simulink model "MSDR_v1"  (R2018a)
settings: Solver=ode23tb  StartTime=0.0  StopTime=50000  RelTol=1e-3
values from neighbouring files (symbols this model uses):
  a_f = -3.22E-5    (= -3.22e-05)    [MSDR_parameters.m]
  a_g = +2.35E-5    (= 2.35e-05)    [MSDR_parameters.m]
  beta = [0.000223, 0.001457, 0.001307, 0.002628, 0.000766, 0.000280]    [MSDR_parameters.m]
  beta_t = sum(beta)    [MSDR_parameters.m]
  Cp_s_shx = 1549.12e-6    (= 0.00154912)    [MSDR_parameters.m]
  Cst = 10    [MSDR_parameters.m]
  dLb = 0    [MSDR_parameters.m]
  dLs = 0    [MSDR_parameters.m]
  dLsc = 0    [MSDR_parameters.m]
  gamma_I = 5.1135e-2    (= 0.051135)    [MSDR_parameters.m]
  gamma_Xe = 1.1628e-2    (= 0.011628)    [MSDR_parameters.m]
  hA_fg = [h_fg*A_fg/2, h_fg*A_fg/2]    [MSDR_parameters.m]
  hA_p_phx1 = h_p_phx*A_p_phx    [MSDR_parameters.m]
  hA_p_phx2 = h_p_phx*A_p_phx    [MSDR_parameters.m]
  hA_p_phx3 = h_p_phx*A_p_phx    [MSDR_parameters.m]
  hA_p_phx4 = h_p_phx*A_p_phx    [MSDR_parameters.m]
  hA_p_phx5 = h_p_phx*A_p_phx    [MSDR_parameters.m]
  hA_p_phx6 = h_p_phx*A_p_phx    [MSDR_parameters.m]
  hA_p_shx1 = h_p_shx*A_p_shx    [MSDR_parameters.m]
  hA_p_shx2 = h_p_shx*A_p_shx    [MSDR_parameters.m]
  hA_p_shx3 = h_p_shx*A_p_shx    [MSDR_parameters.m]
  hA_p_shx4 = h_p_shx*A_p_shx    [MSDR_parameters.m]
  hA_p_shx5 = h_p_shx*A_p_shx    [MSDR_parameters.m]
  hA_p_shx6 = h_p_shx*A_p_shx    [MSDR_parameters.m]
  hA_s_phx1 = h_s_phx*A_s_phx    [MSDR_parameters.m]
  hA_s_phx2 = h_s_phx*A_s_phx    [MSDR_parameters.m]
  hA_s_phx3 = h_s_phx*A_s_phx    [MSDR_parameters.m]
  hA_s_phx4 = h_s_phx*A_s_phx    [MSDR_parameters.m]
  hA_s_phx5 = h_s_phx*A_s_phx    [MSDR_parameters.m]
  hA_s_phx6 = h_s_phx*A_s_phx    [MSDR_parameters.m]
  hA_s_shx1 = h_s_shx*A_s_shx    [MSDR_parameters.m]
  hA_s_shx2 = h_s_shx*A_s_shx    [MSDR_parameters.m]
  hA_s_shx3 = h_s_shx*A_s_shx    [MSDR_parameters.m]
  hA_s_shx4 = h_s_shx*A_s_shx    [MSDR_parameters.m]
  hA_s_shx5 = h_s_shx*A_s_shx    [MSDR_parameters.m]
  hA_s_shx6 = h_s_shx*A_s_shx    [MSDR_parameters.m]
  I_0 = gamma_I*Sig_f_msdr*phi_0/lam_I    (= 4.38204721773e+16)    [MSDR_parameters.m]
  Ifa = [0.25, 0.25]    [MSDR_parameters.m]
  Ifb = [0.25, 0.25]    [MSDR_parameters.m]
  Ig = [0.5, 0.5]    [MSDR_parameters.m]
  J = 1e-6    (= 1e-06)    [MSDR_parameters.m]
  ka = [0.235, 0.235]    [MSDR_parameters.m]
  kb = [0.235, 0.235]    [MSDR_parameters.m]
  kc = 5    [MSDR_parameters.m]
  kga = [0.015, 0.015]    [MSDR_parameters.m]
  kgb = [0.015, 0.015]    [MSDR_parameters.m]
  L = 8.5344    [MSDR_parameters.m]
  Lam = 2.400E-04    (= 0.00024)    [MSDR_parameters.m]
  lam = [0.0124, 0.0305, 0.111, 0.301, 1.14, 3.01]    [MSDR_parameters.m]
  lam_bubl = 2.0e-2    (= 0.02)    [MSDR_parameters.m]
  lam_I = 2.875e-5    (= 2.875e-05)    [MSDR_parameters.m]
  lam_Xe = 2.0916e-5    (= 2.0916e-05)    [MSDR_parameters.m]
  m_3m = W_3*2    (= 8618.207327)    [MSDR_parameters.m]
  m_fm = W_f*2    (= 9978.96)    [MSDR_parameters.m]
  m_sb = 1717    [MSDR_parameters.m]
  mb_cpb = 2.689619410657651e+00    (= 2.68961941066)    [MSDR_parameters.m]
  mcp_fa = mfa*Cp_f    [MSDR_parameters.m]
  mcp_fb = mfb*Cp_f    [MSDR_parameters.m]
  mcp_g = mg*Cp_g    [MSDR_parameters.m]
  mcp_p_phx1 = Cp_p_phx*mp_phx1    [MSDR_parameters.m]
  mcp_p_phx2 = Cp_p_phx*mp_phx2    [MSDR_parameters.m]
  mcp_p_phx3 = Cp_p_phx*mp_phx3    [MSDR_parameters.m]
  mcp_p_phx4 = Cp_p_phx*mp_phx4    [MSDR_parameters.m]
  mcp_p_phx5 = Cp_p_phx*mp_phx5    [MSDR_parameters.m]
  mcp_p_phx6 = Cp_p_phx*mp_phx6    [MSDR_parameters.m]
  mcp_p_shx1 = Cp_p_shx*mp_shx1    [MSDR_parameters.m]
  mcp_p_shx2 = Cp_p_shx*mp_shx2    [MSDR_parameters.m]
  mcp_p_shx3 = Cp_p_shx*mp_shx3    [MSDR_parameters.m]
  mcp_p_shx4 = Cp_p_shx*mp_shx4    [MSDR_parameters.m]
  mcp_p_shx5 = Cp_p_shx*mp_shx5    [MSDR_parameters.m]
  mcp_p_shx6 = Cp_p_shx*mp_shx6    [MSDR_parameters.m]
  mcp_s_phx1 = Cp_s_phx*ms_phx1    [MSDR_parameters.m]
  mcp_s_phx2 = Cp_s_phx*ms_phx2    [MSDR_parameters.m]
  mcp_s_phx3 = Cp_s_phx*ms_phx3    [MSDR_parameters.m]
  mcp_s_phx4 = Cp_s_phx*ms_phx4    [MSDR_parameters.m]
  mcp_s_phx5 = Cp_s_phx*ms_phx5    [MSDR_parameters.m]
  mcp_s_phx6 = Cp_s_phx*ms_phx6    [MSDR_parameters.m]
  mcp_s_shx1 = Cp_s_shx*ms_shx1    [MSDR_parameters.m]
  mcp_s_shx2 = Cp_s_shx*ms_shx1    [MSDR_parameters.m]
  mcp_s_shx3 = Cp_s_shx*ms_shx1    [MSDR_parameters.m]
  mcp_s_shx4 = Cp_s_shx*ms_shx1    [MSDR_parameters.m]
  mcp_s_shx5 = Cp_s_shx*ms_shx1    [MSDR_parameters.m]
  mcp_s_shx6 = Cp_s_shx*ms_shx1    [MSDR_parameters.m]
  mcp_t_phx1 = Cp_t_phx*mt_phx1    [MSDR_parameters.m]
  mcp_t_phx2 = Cp_t_phx*mt_phx2    [MSDR_parameters.m]
  mcp_t_phx3 = Cp_t_phx*mt_phx3    [MSDR_parameters.m]
  mcp_t_phx4 = Cp_t_phx*mt_phx4    [MSDR_parameters.m]
  mcp_t_phx5 = Cp_t_phx*mt_phx5    [MSDR_parameters.m]
  mcp_t_phx6 = Cp_t_phx*mt_phx6    [MSDR_parameters.m]
  mcp_t_shx1 = Cp_t_phx*mt_shx1    [MSDR_parameters.m]
  mcp_t_shx2 = Cp_t_phx*mt_shx2    [MSDR_parameters.m]
  mcp_t_shx3 = Cp_t_phx*mt_shx3    [MSDR_parameters.m]
  mcp_t_shx4 = Cp_t_phx*mt_shx4    [MSDR_parameters.m]
  mcp_t_shx5 = Cp_t_phx*mt_shx5    [MSDR_parameters.m]
  mcp_t_shx6 = Cp_t_phx*mt_shx6    [MSDR_parameters.m]
  mfa = [mass_fn, mass_fn]    [MSDR_parameters.m]
  mfb = [mass_fn, mass_fn]    [MSDR_parameters.m]
  mp_phx1 = [494.7, 494.7, 494.7, 494.7]    [MSDR_parameters.m]
  mp_phx2 = [494.7, 494.7, 494.7, 494.7]    [MSDR_parameters.m]
  mp_phx3 = [494.7, 494.7, 494.7, 494.7]    [MSDR_parameters.m]
  mp_phx4 = [494.7, 494.7, 494.7, 494.7]    [MSDR_parameters.m]
  mp_phx5 = [494.7, 494.7, 494.7, 494.7]    [MSDR_parameters.m]
  mp_phx6 = [494.7, 494.7, 494.7, 494.7]    [MSDR_parameters.m]
  mp_phxm = (Wp_phx1 + Wp_phx2)*1    (= 1663.16)    [MSDR_parameters.m]
  mp_shx1 = [429.3, 429.3, 429.3, 429.3]    [MSDR_parameters.m]
  mp_shx2 = [429.3, 429.3, 429.3, 429.3]    [MSDR_parameters.m]
  mp_shx3 = [429.3, 429.3, 429.3, 429.3]    [MSDR_parameters.m]
  mp_shx4 = [429.3, 429.3, 429.3, 429.3]    [MSDR_parameters.m]
  mp_shx5 = [429.3, 429.3, 429.3, 429.3]    [MSDR_parameters.m]
  mp_shx6 = [429.3, 429.3, 429.3, 429.3]    [MSDR_parameters.m]
  mp_shxm = (Wp_shx1 + Wp_shx2)*1    (= 932.38)    [MSDR_parameters.m]
  ms_phx1 = [1152.5, 1152.5, 1152.5, 1152.5]    [MSDR_parameters.m]
  ms_phx2 = [1152.5, 1152.5, 1152.5, 1152.5]    [MSDR_parameters.m]
  ms_phx3 = [1152.5, 1152.5, 1152.5, 1152.5]    [MSDR_parameters.m]
  ms_phx4 = [1152.5, 1152.5, 1152.5, 1152.5]    [MSDR_parameters.m]
  ms_phx5 = [1152.5, 1152.5, 1152.5, 1152.5]    [MSDR_parameters.m]
  ms_phx6 = [1152.5, 1152.5, 1152.5, 1152.5]    [MSDR_parameters.m]
  ms_phxm = (Ws_phx1 + Ws_phx2)*1    (= 932.38)    [MSDR_parameters.m]
  ms_shx1 = [1861.5, 1861.5, 1861.5, 1861.5]    [MSDR_parameters.m]
  ms_shx2 = [1861.5, 1861.5, 1861.5, 1861.5]    [MSDR_parameters.m]
  ... (+104 more)
undefined symbols (not defined in the file or in its folder): Ak2, As, C0, Cpp, Cps, Cpsc, Cpw, Dit, Dot, hA_p_thx1, hA_p_thx2, hA_p_thx3, hA_s_thx1, hA_s_thx2, hA_s_thx3, hc0, hfg, hfw0, HFW1, hfw10, HFW2, hpw, Hr, hr0, hwb, hws, hwsc, K3, KBHP, KBLP, Lsc, mcp_p_thx1, mcp_p_thx2, mcp_p_thx3, mcp_s_thx1, mcp_s_thx2, mcp_s_thx3, mcp_t_thx1, mcp_t_thx2, mcp_t_thx3, mp_thx1, mp_thx2, mp_thx3, ms_thx1, ms_thx2, ms_thx3, Mstm, nuf, Pp2, Pp3, Pp4, Pp5
libraries: simulink x20, aerolibconvert2 x2
(part 4 of 7)

== system MSDR_v1/HEAT EXCHANGERS/HEAT EXCHANGER LOOP 2/PHX3 HEAT TRANSFER ==
  PRIMARY FLUID INLET TEMPERATURE : Inport
  SECONDARY FLUID INLET TEMPERATURE : Inport  Port=2
  PRIMARY FLOW FRACTION : Inport  Port=3
  PRIMARY HEAT TRANSFER FRACTION : Inport  Port=4
  SECONDARY FLOW FRACTION : Inport  Port=5
  SECONDARY HEAT TRANSFER FRACTION : Inport  Port=6
  Mux : Mux  Inputs=16
      settings: DisplayOption=signals
  To Workspace : ToWorkspace  VariableName=phx3_ht  SampleTime=-1
  Tp1_phx3 : Integrator  InitialCondition=T0_p_phx3(1)
  Tp2_phx3 : Integrator  InitialCondition=T0_p_phx3(2)
  "Tp3_phx3 " : Integrator  InitialCondition=T0_p_phx3(3)
  Tp4_phx3 : Integrator  InitialCondition=T0_p_phx3(4)
  Ts1_phx3 : Integrator  InitialCondition=T0_s_phx3(1)
  Ts2_phx3 : Integrator  InitialCondition=T0_s_phx3(2)
  Ts3_phx3 : Integrator  InitialCondition=T0_s_phx3(3)
  Ts4_phx3 : Integrator  InitialCondition=T0_s_phx3(4)
  Tt1_phx3 : Integrator  InitialCondition=T0_t_phx3(1)
  Tt2_phx3 : Integrator  InitialCondition=T0_t_phx3(2)
  d(Tp1_phx3)/dt : Fcn  Expr=(u[13]*Wp_phx3/mp_phx3(1))*(u[1] - u[3]) + (u[14]*hA_p_phx3(1)/mcp_p_phx3(1))*(u[7] - u[3])
  d(Tp2_phx3)/dt : Fcn  Expr=(u[13]*Wp_phx3/mp_phx3(2))*(u[3] - u[4]) + (u[14]*hA_p_phx3(2)/mcp_p_phx3(2))*(u[7] - u[3])
  d(Tp3_phx3)/dt : Fcn  Expr=(u[13]*Wp_phx3/mp_phx3(3))*(u[4] - u[5]) + (u[14]*hA_p_phx3(3)/mcp_p_phx3(3))*(u[8] - u[5])
  d(Tp4_phx3)/dt : Fcn  Expr=(u[13]*Wp_phx3/mp_phx3(4))*(u[5] - u[6]) + (u[14]*hA_p_phx3(4)/mcp_p_phx3(4))*(u[8] - u[5])
  d(Ts1_phx3)/dt : Fcn  Expr=(u[15]*Ws_phx3/ms_phx3(1))*(u[2] - u[9]) + (u[16]*hA_s_phx3(1)/mcp_s_phx3(1))*(u[8] - u[9])
  d(Ts2_phx3)/dt : Fcn  Expr=(u[15]*Ws_phx3/ms_phx3(2))*(u[9] - u[10]) + (u[16]*hA_s_phx3(2)/mcp_s_phx3(2))*(u[8] - u[9])
  d(Ts3_phx3)/dt : Fcn  Expr=(u[15]*Ws_phx3/ms_phx3(3))*(u[10] - u[11]) + (u[16]*hA_s_phx3(3)/mcp_s_phx3(3))*(u[7] - u[11])
  d(Ts4_phx3)/dt : Fcn  Expr=(u[15]*Ws_phx3/ms_phx3(4))*(u[11] - u[12]) + (u[16]*hA_s_phx3(4)/mcp_s_phx3(4))*(u[7] - u[11])
  d(Tt1_phx3)/dt : Fcn  Expr=(u[14]*(hA_p_phx3(1) + hA_p_phx3(2))/mcp_t_phx3(1))*(u[3] - u[7]) + (u[16]*(hA_s_phx3(1) + hA_s_phx3(2))/mcp_t_phx3(1))*(u[11] - u[7])
  d(Tt2_phx3)/dt : Fcn  Expr=(u[14]*(hA_p_phx3(3) + hA_p_phx3(4))/mcp_t_phx3(2))*(u[5] - u[8]) + (u[16]*(hA_s_phx3(3) + hA_s_phx3(4))/mcp_t_phx3(2))*(u[9] - u[8])
  PHX3 TEMPERATURES : Outport
  wires:
  Ts1_phx3/1 -> Mux/9
  Ts2_phx3/1 -> Mux/10
  d(Ts2_phx3)/dt/1 -> Ts2_phx3/1
  d(Tp4_phx3)/dt/1 -> Tp4_phx3/1
  Tt1_phx3/1 -> Mux/7
  d(Tp2_phx3)/dt/1 -> Tp2_phx3/1
  Tp4_phx3/1 -> Mux/6
  d(Tt2_phx3)/dt/1 -> Tt2_phx3/1
  SECONDARY FLUID INLET TEMPERATURE/1 -> Mux/2
  Tt2_phx3/1 -> Mux/8
  Mux/1 -> To Workspace/1, PHX3 TEMPERATURES/1, d(Ts4_phx3)/dt/1, d(Ts3_phx3)/dt/1, d(Ts1_phx3)/dt/1, d(Tt2_phx3)/dt/1, d(Tt1_phx3)/dt/1, d(Tp4_phx3)/dt/1, d(Tp3_phx3)/dt/1, d(Tp2_phx3)/dt/1, d(Tp1_phx3)/dt/1, d(Ts2_phx3)/dt/1
  d(Tp1_phx3)/dt/1 -> Tp1_phx3/1
  d(Ts4_phx3)/dt/1 -> Ts4_phx3/1
  Tp1_phx3/1 -> Mux/3
  d(Ts1_phx3)/dt/1 -> Ts1_phx3/1
  d(Ts3_phx3)/dt/1 -> Ts3_phx3/1
  Ts3_phx3/1 -> Mux/11
  Ts4_phx3/1 -> Mux/12
  "Tp3_phx3 "/1 -> Mux/5
  d(Tp3_phx3)/dt/1 -> "Tp3_phx3 "/1
  Tp2_phx3/1 -> Mux/4
  d(Tt1_phx3)/dt/1 -> Tt1_phx3/1
  PRIMARY FLUID INLET TEMPERATURE/1 -> Mux/1
  PRIMARY FLOW FRACTION/1 -> Mux/13
  PRIMARY HEAT TRANSFER FRACTION/1 -> Mux/14
  SECONDARY FLOW FRACTION/1 -> Mux/15
  SECONDARY HEAT TRANSFER FRACTION/1 -> Mux/16

== system MSDR_v1/HEAT EXCHANGERS/HEAT EXCHANGER LOOP 2/PHX3 MATERIAL TRANSPORT ==
  PHX3 TEMPERATURES : Inport
  wires:
  PHX3 TEMPERATURES/1 -> ?

== system MSDR_v1/HEAT EXCHANGERS/HEAT EXCHANGER LOOP 2/PHX4 HEAT TRANSFER ==
  PRIMARY FLUID INLET TEMPERATURE : Inport
  SECONDARY FLUID INLET TEMPERATURE : Inport  Port=2
  PRIMARY FLOW FRACTION : Inport  Port=3
  PRIMARY HEAT TRANSFER FRACTION : Inport  Port=4
  SECONDARY FLOW FRACTION : Inport  Port=5
  SECONDARY HEAT TRANSFER FRACTION : Inport  Port=6
  Mux : Mux  Inputs=16
      settings: DisplayOption=signals
  To Workspace : ToWorkspace  VariableName=phx4_ht  SampleTime=-1
  Tp1_phx4 : Integrator  InitialCondition=T0_p_phx4(1)
  Tp2_phx4 : Integrator  InitialCondition=T0_p_phx4(2)
  "Tp3_phx4 " : Integrator  InitialCondition=T0_p_phx4(3)
  Tp4_phx4 : Integrator  InitialCondition=T0_p_phx4(4)
  Ts1_phx4 : Integrator  InitialCondition=T0_s_phx4(1)
  Ts2_phx4 : Integrator  InitialCondition=T0_s_phx4(2)
  Ts3_phx4 : Integrator  InitialCondition=T0_s_phx4(3)
  Ts4_phx4 : Integrator  InitialCondition=T0_s_phx4(4)
  Tt1_phx4 : Integrator  InitialCondition=T0_t_phx4(1)
  Tt2_phx4 : Integrator  InitialCondition=T0_t_phx4(2)
  d(Tp1_phx4)/dt : Fcn  Expr=(u[13]*Wp_phx4/mp_phx4(1))*(u[1] - u[3]) + (u[14]*hA_p_phx4(1)/mcp_p_phx4(1))*(u[7] - u[3])
  d(Tp2_phx4)/dt : Fcn  Expr=(u[13]*Wp_phx4/mp_phx4(2))*(u[3] - u[4]) + (u[14]*hA_p_phx4(2)/mcp_p_phx4(2))*(u[7] - u[3])
  d(Tp3_phx4)/dt : Fcn  Expr=(u[13]*Wp_phx4/mp_phx4(3))*(u[4] - u[5]) + (u[14]*hA_p_phx4(3)/mcp_p_phx4(3))*(u[8] - u[5])
  d(Tp4_phx4)/dt : Fcn  Expr=(u[13]*Wp_phx4/mp_phx4(4))*(u[5] - u[6]) + (u[14]*hA_p_phx4(4)/mcp_p_phx4(4))*(u[8] - u[5])
  d(Ts1_phx4)/dt : Fcn  Expr=(u[15]*Ws_phx4/ms_phx4(1))*(u[2] - u[9]) + (u[16]*hA_s_phx4(1)/mcp_s_phx4(1))*(u[8] - u[9])
  d(Ts2_phx4)/dt : Fcn  Expr=(u[15]*Ws_phx4/ms_phx4(2))*(u[9] - u[10]) + (u[16]*hA_s_phx4(2)/mcp_s_phx4(2))*(u[8] - u[9])
  d(Ts3_phx4)/dt : Fcn  Expr=(u[15]*Ws_phx4/ms_phx4(3))*(u[10] - u[11]) + (u[16]*hA_s_phx4(3)/mcp_s_phx4(3))*(u[7] - u[11])
  d(Ts4_phx4)/dt : Fcn  Expr=(u[15]*Ws_phx4/ms_phx4(4))*(u[11] - u[12]) + (u[16]*hA_s_phx4(4)/mcp_s_phx4(4))*(u[7] - u[11])
  d(Tt1_phx4)/dt : Fcn  Expr=(u[14]*(hA_p_phx4(1) + hA_p_phx4(2))/mcp_t_phx4(1))*(u[3] - u[7]) + (u[16]*(hA_s_phx4(1) + hA_s_phx4(2))/mcp_t_phx4(1))*(u[11] - u[7])
  d(Tt2_phx4)/dt : Fcn  Expr=(u[14]*(hA_p_phx4(3) + hA_p_phx4(4))/mcp_t_phx4(2))*(u[5] - u[8]) + (u[16]*(hA_s_phx4(3) + hA_s_phx4(4))/mcp_t_phx4(2))*(u[9] - u[8])
  PHX4 TEMPERATURES : Outport
  wires:
  Ts1_phx4/1 -> Mux/9
  Ts2_phx4/1 -> Mux/10
  d(Ts2_phx4)/dt/1 -> Ts2_phx4/1
  d(Tp4_phx4)/dt/1 -> Tp4_phx4/1
  Tt1_phx4/1 -> Mux/7
  d(Tp2_phx4)/dt/1 -> Tp2_phx4/1
  Tp4_phx4/1 -> Mux/6
  d(Tt2_phx4)/dt/1 -> Tt2_phx4/1
  SECONDARY FLUID INLET TEMPERATURE/1 -> Mux/2
  Tt2_phx4/1 -> Mux/8
  Mux/1 -> To Workspace/1, PHX4 TEMPERATURES/1, d(Ts4_phx4)/dt/1, d(Ts3_phx4)/dt/1, d(Ts1_phx4)/dt/1, d(Tt2_phx4)/dt/1, d(Tt1_phx4)/dt/1, d(Tp4_phx4)/dt/1, d(Tp3_phx4)/dt/1, d(Tp2_phx4)/dt/1, d(Tp1_phx4)/dt/1, d(Ts2_phx4)/dt/1
  d(Tp1_phx4)/dt/1 -> Tp1_phx4/1
  d(Ts4_phx4)/dt/1 -> Ts4_phx4/1
  Tp1_phx4/1 -> Mux/3
  d(Ts1_phx4)/dt/1 -> Ts1_phx4/1
  d(Ts3_phx4)/dt/1 -> Ts3_phx4/1
  Ts3_phx4/1 -> Mux/11
  Ts4_phx4/1 -> Mux/12
  "Tp3_phx4 "/1 -> Mux/5
  d(Tp3_phx4)/dt/1 -> "Tp3_phx4 "/1
  Tp2_phx4/1 -> Mux/4
  d(Tt1_phx4)/dt/1 -> Tt1_phx4/1
  PRIMARY FLUID INLET TEMPERATURE/1 -> Mux/1
  PRIMARY FLOW FRACTION/1 -> Mux/13
  PRIMARY HEAT TRANSFER FRACTION/1 -> Mux/14
  SECONDARY FLOW FRACTION/1 -> Mux/15
  SECONDARY HEAT TRANSFER FRACTION/1 -> Mux/16

== system MSDR_v1/HEAT EXCHANGERS/HEAT EXCHANGER LOOP 2/PHX4 MATERIAL TRANSPORT ==
  PHX4 TEMPERATURES : Inport
  wires:
  PHX4 TEMPERATURES/1 -> ?

== system MSDR_v1/HEAT EXCHANGERS/HEAT EXCHANGER LOOP 2/SHX PRIM MIXING ==
  Tp_shx3 : Inport
  Tp_shx4 : Inport  Port=2
  p_flow_frac : Inport  Port=3
  Fcn : Fcn  Expr=u[3]*Wp_shx3/mp_shxm*(u[1]-u[4]) + u[3]*Wp_shx4/mp_shxm*(u[2]-u[4])
  Integrator : Integrator  InitialCondition=T0_p_shx1(4)
  Mux : Mux
  Tp_shx_mix : Outport
  wires:
  Tp_shx3/1 -> Mux/1
  Tp_shx4/1 -> Mux/2
  Mux/1 -> Fcn/1
  p_flow_frac/1 -> Mux/3
  Fcn/1 -> Integrator/1
  Integrator/1 -> Tp_shx_mix/1, Mux/4

== system MSDR_v1/HEAT EXCHANGERS/HEAT EXCHANGER LOOP 2/SHX SEC MIXING ==
  Ts_shx3 : Inport
  Ts_shx4 : Inport  Port=2
  s_flow_frac : Inport  Port=3
  Fcn : Fcn  Expr=u[3]*Ws_shx3/ms_shxm*(u[1]-u[4]) + u[3]*Ws_shx4/ms_shxm*(u[2]-u[4])
  Integrator : Integrator  InitialCondition=T0_s_shx1(4)
  Mux : Mux
  Ts_shx_mix : Outport
  wires:
  Ts_shx3/1 -> Mux/1
  Ts_shx4/1 -> Mux/2
  Mux/1 -> Fcn/1
  s_flow_frac/1 -> Mux/3
  Fcn/1 -> Integrator/1
  Integrator/1 -> Ts_shx_mix/1, Mux/4

== system MSDR_v1/HEAT EXCHANGERS/HEAT EXCHANGER LOOP 2/SHX//THX PUMP ==
  1-D Lookup Table : Lookup_n-D  NumberOfTableDimensions=1  BreakpointsForDimension1=xdat  Table=ydat  InternalRulePriority=Speed  RndMeth=Simplest  InputSameDT=on
  Clock : Clock
  Fcn : Fcn  Expr=exp((1/tau_p)*u)
  Final convection flow rate : Constant  Value=therm_conv
  Scope : Scope
  Subtract : Sum  Inputs=-+
  Switch : Switch  Criteria=u2 > Threshold
  Transport Delay : TransportDelay  DelayTime=20000000  InitialOutput=1
  FLOW FRACTION : Outport
  HEAT TRANSFER FRACTION : Outport  Port=2
  wires:
  Transport Delay/1 -> 1-D Lookup Table/1, Scope/1, FLOW FRACTION/1
  Clock/1 -> Fcn/1
  Switch/1 -> Transport Delay/1
  Fcn/1 -> Subtract/1, Switch/1
  Final convection flow rate/1 -> Subtract/2, Switch/3
  Subtract/1 -> Switch/2
  1-D Lookup Table/1 -> HEAT TRANSFER FRACTION/1

== system MSDR_v1/HEAT EXCHANGERS/HEAT EXCHANGER LOOP 2/SHX3 HEAT TRANSFER ==
  PRIMARY FLUID INLET TEMPERATURE : Inport
  SECONDARY FLUID INLET TEMPERATURE : Inport  Port=2
  PRIMARY FLOW FRACTION : Inport  Port=3
  PRIMARY HEAT TRANSFER FRACTION : Inport  Port=4
  SECONDARY FLOW FRACTION : Inport  Port=5
  SECONDARY HEAT TRANSFER FRACTION : Inport  Port=6
  Mux : Mux  Inputs=16
      settings: DisplayOption=signals
  To Workspace : ToWorkspace  VariableName=shx3_ht  SampleTime=-1
  Tp1_shx3 : Integrator  InitialCondition=T0_p_shx3(1)
  Tp2_shx3 : Integrator  InitialCondition=T0_p_shx3(2)
  "Tp3_shx3 " : Integrator  InitialCondition=T0_p_shx3(3)
  Tp4_shx3 : Integrator  InitialCondition=T0_p_shx3(4)
  Ts1_shx3 : Integrator  InitialCondition=T0_s_shx3(1)
  Ts2_shx3 : Integrator  InitialCondition=T0_s_shx3(2)
  Ts3_shx3 : Integrator  InitialCondition=T0_s_shx3(3)
  Ts4_shx3 : Integrator  InitialCondition=T0_s_shx3(4)
  Tt1_shx3 : Integrator  InitialCondition=T0_t_shx3(1)
  Tt2_shx3 : Integrator  InitialCondition=T0_t_shx3(2)
  d(Tp1_shx3)/dt : Fcn  Expr=(u[13]*Wp_shx3/mp_shx3(1))*(u[1] - u[3]) + (u[14]*hA_p_shx3(1)/mcp_p_shx3(1))*(u[7] - u[3])
  d(Tp2_shx3)/dt : Fcn  Expr=(u[13]*Wp_shx3/mp_shx3(2))*(u[3] - u[4]) + (u[14]*hA_p_shx3(2)/mcp_p_shx3(2))*(u[7] - u[3])
  d(Tp3_shx3)/dt : Fcn  Expr=(u[13]*Wp_shx3/mp_shx3(3))*(u[4] - u[5]) + (u[14]*hA_p_shx3(3)/mcp_p_shx3(3))*(u[8] - u[5])
  d(Tp4_shx3)/dt : Fcn  Expr=(u[13]*Wp_shx3/mp_shx3(4))*(u[5] - u[6]) + (u[14]*hA_p_shx3(4)/mcp_p_shx3(4))*(u[8] - u[5])
  d(Ts1_shx3)/dt : Fcn  Expr=(u[15]*Ws_shx3/ms_shx3(1))*(u[2] - u[9]) + (u[16]*hA_s_shx3(1)/mcp_s_shx3(1))*(u[8] - u[9])
  d(Ts2_shx3)/dt : Fcn  Expr=(u[15]*Ws_shx3/ms_shx3(2))*(u[9] - u[10]) + (u[16]*hA_s_shx3(2)/mcp_s_shx3(2))*(u[8] - u[9])
  d(Ts3_shx3)/dt : Fcn  Expr=(u[15]*Ws_shx3/ms_shx3(3))*(u[10] - u[11]) + (u[16]*hA_s_shx3(3)/mcp_s_shx3(3))*(u[7] - u[11])
  d(Ts4_shx3)/dt : Fcn  Expr=(u[15]*Ws_shx3/ms_shx3(4))*(u[11] - u[12]) + (u[16]*hA_s_shx3(4)/mcp_s_shx3(4))*(u[7] - u[11])
  d(Tt1_shx3)/dt : Fcn  Expr=(u[14]*(hA_p_shx3(1) + hA_p_shx3(2))/mcp_t_shx3(1))*(u[3] - u[7]) + (u[16]*(hA_s_shx3(1) + hA_s_shx3(2))/mcp_t_shx3(1))*(u[11] - u[7])
  d(Tt2_shx3)/dt : Fcn  Expr=(u[14]*(hA_p_shx4(3) + hA_p_shx4(4))/mcp_t_shx4(2))*(u[5] - u[8]) + (u[16]*(hA_s_shx4(3) + hA_s_shx4(4))/mcp_t_shx4(2))*(u[9] - u[8])
  SHX3 TEMPERATURES : Outport
  wires:
  Ts1_shx3/1 -> Mux/9
  Ts2_shx3/1 -> Mux/10
  d(Ts2_shx3)/dt/1 -> Ts2_shx3/1
  d(Tp4_shx3)/dt/1 -> Tp4_shx3/1
  Tt1_shx3/1 -> Mux/7
  d(Tp2_shx3)/dt/1 -> Tp2_shx3/1
  Tp4_shx3/1 -> Mux/6
  d(Tt2_shx3)/dt/1 -> Tt2_shx3/1
  SECONDARY FLUID INLET TEMPERATURE/1 -> Mux/2
  Tt2_shx3/1 -> Mux/8
  Mux/1 -> To Workspace/1, SHX3 TEMPERATURES/1, d(Ts4_shx3)/dt/1, d(Ts3_shx3)/dt/1, d(Ts2_shx3)/dt/1, d(Ts1_shx3)/dt/1, d(Tt2_shx3)/dt/1, d(Tt1_shx3)/dt/1, d(Tp4_shx3)/dt/1, d(Tp3_shx3)/dt/1, d(Tp2_shx3)/dt/1, d(Tp1_shx3)/dt/1
  d(Tp1_shx3)/dt/1 -> Tp1_shx3/1
  d(Ts4_shx3)/dt/1 -> Ts4_shx3/1
  Tp1_shx3/1 -> Mux/3
  d(Ts1_shx3)/dt/1 -> Ts1_shx3/1
  d(Ts3_shx3)/dt/1 -> Ts3_shx3/1
  Ts3_shx3/1 -> Mux/11
  Ts4_shx3/1 -> Mux/12
  "Tp3_shx3 "/1 -> Mux/5
  d(Tp3_shx3)/dt/1 -> "Tp3_shx3 "/1
  Tp2_shx3/1 -> Mux/4
  d(Tt1_shx3)/dt/1 -> Tt1_shx3/1
  PRIMARY FLUID INLET TEMPERATURE/1 -> Mux/1
  PRIMARY FLOW FRACTION/1 -> Mux/13
  PRIMARY HEAT TRANSFER FRACTION/1 -> Mux/14
  SECONDARY FLOW FRACTION/1 -> Mux/15
  SECONDARY HEAT TRANSFER FRACTION/1 -> Mux/16

== system MSDR_v1/HEAT EXCHANGERS/HEAT EXCHANGER LOOP 2/SHX3 MATERIAL TRANSPORT ==
  SHX3 TEMPERATURES : Inport
  wires:
  SHX3 TEMPERATURES/1 -> ?

== system MSDR_v1/HEAT EXCHANGERS/HEAT EXCHANGER LOOP 2/SHX4 HEAT TRANSFER ==
  PRIMARY FLUID INLET TEMPERATURE : Inport
  SECONDARY FLUID INLET TEMPERATURE : Inport  Port=2
  PRIMARY FLOW FRACTION : Inport  Port=3
  PRIMARY HEAT TRANSFER FRACTION : Inport  Port=4
  SECONDARY FLOW FRACTION : Inport  Port=5
  SECONDARY HEAT TRANSFER FRACTION : Inport  Port=6
  Mux : Mux  Inputs=16
      settings: DisplayOption=signals
  To Workspace : ToWorkspace  VariableName=shx4_ht  SampleTime=-1
  Tp1_shx4 : Integrator  InitialCondition=T0_p_shx4(1)
  Tp2_shx4 : Integrator  InitialCondition=T0_p_shx4(2)
  "Tp3_shx4 " : Integrator  InitialCondition=T0_p_shx4(3)
  Tp4_shx4 : Integrator  InitialCondition=T0_p_shx4(4)
  Ts1_shx4 : Integrator  InitialCondition=T0_s_shx4(1)
  Ts2_shx4 : Integrator  InitialCondition=T0_s_shx4(2)
  Ts3_shx4 : Integrator  InitialCondition=T0_s_shx4(3)
  Ts4_shx4 : Integrator  InitialCondition=T0_s_shx4(4)
  Tt1_shx4 : Integrator  InitialCondition=T0_t_shx4(1)
  Tt2_shx4 : Integrator  InitialCondition=T0_t_shx4(2)
  d(Tp1_shx4)/dt : Fcn  Expr=(u[13]*Wp_shx4/mp_shx4(1))*(u[1] - u[3]) + (u[14]*hA_p_shx4(1)/mcp_p_shx4(1))*(u[7] - u[3])
  d(Tp2_shx4)/dt : Fcn  Expr=(u[13]*Wp_shx4/mp_shx4(2))*(u[3] - u[4]) + (u[14]*hA_p_shx4(2)/mcp_p_shx4(2))*(u[7] - u[3])
  d(Tp3_shx4)/dt : Fcn  Expr=(u[13]*Wp_shx4/mp_shx4(3))*(u[4] - u[5]) + (u[14]*hA_p_shx4(3)/mcp_p_shx4(3))*(u[8] - u[5])
  d(Tp4_shx4)/dt : Fcn  Expr=(u[13]*Wp_shx4/mp_shx4(4))*(u[5] - u[6]) + (u[14]*hA_p_shx4(4)/mcp_p_shx4(4))*(u[8] - u[5])
  d(Ts1_shx4)/dt : Fcn  Expr=(u[15]*Ws_shx4/ms_shx4(1))*(u[2] - u[9]) + (u[16]*hA_s_shx4(1)/mcp_s_shx4(1))*(u[8] - u[9])
  d(Ts2_shx4)/dt : Fcn  Expr=(u[15]*Ws_shx4/ms_shx4(2))*(u[9] - u[10]) + (u[16]*hA_s_shx4(2)/mcp_s_shx4(2))*(u[8] - u[9])
  d(Ts3_shx4)/dt : Fcn  Expr=(u[15]*Ws_shx4/ms_shx4(3))*(u[10] - u[11]) + (u[16]*hA_s_shx4(3)/mcp_s_shx4(3))*(u[7] - u[11])
  d(Ts4_shx4)/dt : Fcn  Expr=(u[15]*Ws_shx4/ms_shx4(4))*(u[11] - u[12]) + (u[16]*hA_s_shx4(4)/mcp_s_shx4(4))*(u[7] - u[11])
  d(Tt1_shx4)/dt : Fcn  Expr=(u[14]*(hA_p_shx4(1) + hA_p_shx4(2))/mcp_t_shx4(1))*(u[3] - u[7]) + (u[16]*(hA_s_shx4(1) + hA_s_shx4(2))/mcp_t_shx4(1))*(u[11] - u[7])
  d(Tt2_shx4)/dt : Fcn  Expr=(u[14]*(hA_p_shx4(3) + hA_p_shx4(4))/mcp_t_shx4(2))*(u[5] - u[8]) + (u[16]*(hA_s_shx4(3) + hA_s_shx4(4))/mcp_t_shx4(2))*(u[9] - u[8])
  SHX4 TEMPERATURES : Outport
  wires:
  Ts1_shx4/1 -> Mux/9
  Ts2_shx4/1 -> Mux/10
  d(Ts2_shx4)/dt/1 -> Ts2_shx4/1
  d(Tp4_shx4)/dt/1 -> Tp4_shx4/1
  Tt1_shx4/1 -> Mux/7
  d(Tp2_shx4)/dt/1 -> Tp2_shx4/1
  Tp4_shx4/1 -> Mux/6
  d(Tt2_shx4)/dt/1 -> Tt2_shx4/1
  SECONDARY FLUID INLET TEMPERATURE/1 -> Mux/2
  Tt2_shx4/1 -> Mux/8
  Mux/1 -> To Workspace/1, SHX4 TEMPERATURES/1, d(Ts4_shx4)/dt/1, d(Ts3_shx4)/dt/1, d(Ts2_shx4)/dt/1, d(Ts1_shx4)/dt/1, d(Tt2_shx4)/dt/1, d(Tt1_shx4)/dt/1, d(Tp4_shx4)/dt/1, d(Tp3_shx4)/dt/1, d(Tp2_shx4)/dt/1, d(Tp1_shx4)/dt/1
  d(Tp1_shx4)/dt/1 -> Tp1_shx4/1
  d(Ts4_shx4)/dt/1 -> Ts4_shx4/1
  Tp1_shx4/1 -> Mux/3
  d(Ts1_shx4)/dt/1 -> Ts1_shx4/1
  d(Ts3_shx4)/dt/1 -> Ts3_shx4/1
  Ts3_shx4/1 -> Mux/11
  Ts4_shx4/1 -> Mux/12
  "Tp3_shx4 "/1 -> Mux/5
  d(Tp3_shx4)/dt/1 -> "Tp3_shx4 "/1
  Tp2_shx4/1 -> Mux/4
  d(Tt1_shx4)/dt/1 -> Tt1_shx4/1
  PRIMARY FLUID INLET TEMPERATURE/1 -> Mux/1
  PRIMARY FLOW FRACTION/1 -> Mux/13
  PRIMARY HEAT TRANSFER FRACTION/1 -> Mux/14
  SECONDARY FLOW FRACTION/1 -> Mux/15
  SECONDARY HEAT TRANSFER FRACTION/1 -> Mux/16

== system MSDR_v1/HEAT EXCHANGERS/HEAT EXCHANGER LOOP 2/SHX4 MATERIAL TRANSPORT ==
  SHX4 TEMPERATURES : Inport
  wires:
  SHX4 TEMPERATURES/1 -> ?

== system MSDR_v1/HEAT EXCHANGERS/HEAT EXCHANGER LOOP 2/THX2 HEAT TRANSFER ==
  PRIMARY FLUID INLET TEMPERATURE : Inport
  SECONDARY FLUID INLET TEMPERATURE : Inport  Port=2
  PRIMARY FLOW FRACTION : Inport  Port=3
  PRIMARY HEAT TRANSFER FRACTION : Inport  Port=4
  SECONDARY FLOW FRACTION : Inport  Port=5
  SECONDARY HEAT TRANSFER FRACTION : Inport  Port=6
  Mux : Mux  Inputs=16
      settings: DisplayOption=signals
  To Workspace : ToWorkspace  VariableName=thx2_ht  SampleTime=-1
  Tp1_thx2 : Integrator  InitialCondition=T0_p_thx2(1)
  Tp2_thx2 : Integrator  InitialCondition=T0_p_thx2(2)
  "Tp3_thx2 " : Integrator  InitialCondition=T0_p_thx2(3)
  Tp4_thx2 : Integrator  InitialCondition=T0_p_thx2(4)
  Ts1_thx2 : Integrator  InitialCondition=T0_s_thx2(1)
  Ts2_thx2 : Integrator  InitialCondition=T0_s_thx2(2)
  Ts3_thx2 : Integrator  InitialCondition=T0_s_thx2(3)
  Ts4_thx2 : Integrator  InitialCondition=T0_s_thx2(4)
  Tt1_thx2 : Integrator  InitialCondition=T0_t_thx2(1)
  Tt2_thx2 : Integrator  InitialCondition=T0_t_thx2(2)
  d(Tp1_thx2)/dt : Fcn  Expr=(u[13]*Wp_thx2/mp_thx2(1))*(u[1] - u[3]) + (u[14]*hA_p_thx2(1)/mcp_p_thx2(1))*(u[7] - u[3])
  d(Tp2_thx2)/dt : Fcn  Expr=(u[13]*Wp_thx2/mp_thx2(2))*(u[3] - u[4]) + (u[14]*hA_p_thx2(2)/mcp_p_thx2(2))*(u[7] - u[3])
  d(Tp3_thx2)/dt : Fcn  Expr=(u[13]*Wp_thx2/mp_thx2(3))*(u[4] - u[5]) + (u14]*hA_p_thx2(3)/mcp_p_thx2(3))*(u[8] - u[5])
  d(Tp4_thx2)/dt : Fcn  Expr=(u[13]*Wp_thx2/mp_thx2(4))*(u[5] - u[6]) + (u[14]*hA_p_thx2(4)/mcp_p_thx2(4))*(u[8] - u[5])
  d(Ts1_thx2)/dt : Fcn  Expr=(u[15]*Ws_thx2/ms_thx2(1))*(u[2] - u[9]) + (u[16]*hA_s_thx2(1)/mcp_s_thx2(1))*(u[8] - u[9])
  d(Ts2_thx2)/dt : Fcn  Expr=(u[15]*Ws_thx2/ms_thx2(2))*(u[9] - u[10]) + (u[16]*hA_s_thx2(2)/mcp_s_thx2(2))*(u[8] - u[9])
  d(Ts3_thx2)/dt : Fcn  Expr=(u[15]*Ws_thx2/ms_thx2(3))*(u[10] - u[11]) + (u[16]*hA_s_thx2(3)/mcp_s_thx2(3))*(u[7] - u[11])
  d(Ts4_thx2)/dt : Fcn  Expr=(u[15]*Ws_thx2/ms_thx2(4))*(u[11] - u[12]) + (u[16]*hA_s_thx2(4)/mcp_s_thx2(4))*(u[7] - u[11])
  d(Tt1_thx2)/dt : Fcn  Expr=(u[14]*(hA_p_thx2(1) + hA_p_thx2(2))/mcp_t_thx2(1))*(u[3] - u[7]) + (u[16]*(hA_s_thx2(1) + hA_s_thx2(2))/mcp_t_thx2(1))*(u[11] - u[7])
  d(Tt2_thx2)/dt : Fcn  Expr=(u[14]*(hA_p_thx2(3) + hA_p_thx2(4))/mcp_t_thx2(2))*(u[5] - u[8]) + (u[16]*(hA_s_thx2(3) + hA_s_thx2(4))/mcp_t_thx2(2))*(u[9] - u[8])
  THX2 TEMPERATURES : Outport
  wires:
  Ts1_thx2/1 -> Mux/9
  Ts2_thx2/1 -> Mux/10
  d(Ts2_thx2)/dt/1 -> Ts2_thx2/1
  d(Tp4_thx2)/dt/1 -> Tp4_thx2/1
  Tt1_thx2/1 -> Mux/7
  d(Tp2_thx2)/dt/1 -> Tp2_thx2/1
  Tp4_thx2/1 -> Mux/6
  d(Tt2_thx2)/dt/1 -> Tt2_thx2/1
  SECONDARY FLUID INLET TEMPERATURE/1 -> Mux/2
  Tt2_thx2/1 -> Mux/8
  Mux/1 -> To Workspace/1, THX2 TEMPERATURES/1, d(Ts4_thx2)/dt/1, d(Ts3_thx2)/dt/1, d(Ts2_thx2)/dt/1, d(Ts1_thx2)/dt/1, d(Tt2_thx2)/dt/1, d(Tt1_thx2)/dt/1, d(Tp4_thx2)/dt/1, d(Tp3_thx2)/dt/1, d(Tp2_thx2)/dt/1, d(Tp1_thx2)/dt/1
  d(Tp1_thx2)/dt/1 -> Tp1_thx2/1
  d(Ts4_thx2)/dt/1 -> Ts4_thx2/1
  Tp1_thx2/1 -> Mux/3
  d(Ts1_thx2)/dt/1 -> Ts1_thx2/1
  d(Ts3_thx2)/dt/1 -> Ts3_thx2/1
  Ts3_thx2/1 -> Mux/11
  Ts4_thx2/1 -> Mux/12
  "Tp3_thx2 "/1 -> Mux/5
  d(Tp3_thx2)/dt/1 -> "Tp3_thx2 "/1
  Tp2_thx2/1 -> Mux/4
  d(Tt1_thx2)/dt/1 -> Tt1_thx2/1
  PRIMARY FLUID INLET TEMPERATURE/1 -> Mux/1
  PRIMARY FLOW FRACTION/1 -> Mux/13
  PRIMARY HEAT TRANSFER FRACTION/1 -> Mux/14
  SECONDARY FLOW FRACTION/1 -> Mux/15
  SECONDARY HEAT TRANSFER FRACTION/1 -> Mux/16

== system MSDR_v1/HEAT EXCHANGERS/HEAT EXCHANGER LOOP 2/THX2 MATERIAL TRANSPORT ==
  THX2 TEMPERATURES : Inport
  wires:
  THX2 TEMPERATURES/1 -> ?

== system MSDR_v1/HEAT EXCHANGERS/HEAT EXCHANGER LOOP 3/BOILER & REHEATER ==
  Coolant Inlet Temp : Inport
  Power Demand (Frac) : Inport  Port=2
  Fcn : Fcn  Commented=on  Expr=u[1] - u[2]*250/((Ws_shx1 + Ws_shx2)*Cp_s_shx)
  Integrator : Integrator  InitialCondition=400
  Mux : Mux  Inputs=3
      settings: DisplayOption=signals
  To Workspace : ToWorkspace  VariableName=msdr_br_mux3  SampleTime=-1
  ddt_t_b = 1/tau_b*(t_bin-t_b)-p_b/mb_cpb : Fcn  Expr=W_sb*(u(1)-u(3))/m_sb - u(2)/mb_cpb
  Coolant Exit Temp : Outport
  wires:
  Coolant Inlet Temp/1 -> Mux/1
  Mux/1 -> ddt_t_b = 1/tau_b*(t_bin-t_b)-p_b/mb_cpb/1, To Workspace/1
  Power Demand (Frac)/1 -> Mux/2
  Integrator/1 -> Coolant Exit Temp/1, Mux/3
  ddt_t_b = 1/tau_b*(t_bin-t_b)-p_b/mb_cpb/1 -> Integrator/1

== system MSDR_v1/HEAT EXCHANGERS/HEAT EXCHANGER LOOP 3/Fractional Power Demand (fractional) ==
  Add : Sum
  Constant : Constant
  Saturation : Saturate  UpperLimit=1  LowerLimit=0.2
  Saturation1 : Saturate  UpperLimit=.8  LowerLimit=0
  Slider : Subsystem  DialogController=hmiCreateDDGDialog  IsWebBlock=on  mask(MWDashboardBlock){webBlockId=9afe0574-93b5-4d2b-9630-def9aae4c12d, webBlockType=slider, ShowInLibBrowser=on, ShowInitialText=on, HMISrcModelName=[]}
      mask prompts: webBlockId "WebBlock Id"; webBlockType "WebBlock Type"; HMISrcModelName "Source Model"
      mask help: SimulinkHMI:dialogs:SliderDialogDesc
      mask Help: helpview([docroot '/mapfiles/simulink.map'], 'hmi_slider')
      mask Display:
      | if strcmp(get_param(bdroot(gcb),'BlockDiagramType'), 'library')
      |     image([(matlabroot) '/toolbox/simulink/hmi/icons/Slider.png']);
      | end
  down 1%/min : simulink/Sources/Ramp  slope=-0.01/60  start=2500  InitialOutput=1
  up 1%/min1 : simulink/Sources/Ramp  slope=0.01/60  start=2500+3600+5000  InitialOutput=0
  Power Demand(frac) : Outport
  wires:
  down 1%/min/1 -> Saturation/1
  Saturation/1 -> Add/1
  up 1%/min1/1 -> Saturation1/1
  Saturation1/1 -> Add/2
  Constant/1 -> Power Demand(frac)/1

== system MSDR_v1/HEAT EXCHANGERS/HEAT EXCHANGER LOOP 3/PHX PRIM MIXING ==
  Tp_phx5 : Inport
  Tp_phx6 : Inport  Port=2
  p_flow_frac : Inport  Port=3
  Fcn : Fcn  Expr=u[3]*Wp_phx5/mp_phxm*(u[1]-u[4]) + u[3]*Wp_phx6/mp_phxm*(u[2]-u[4])
  Integrator : Integrator  InitialCondition=Tf_in
  Mux : Mux
  Tp_phx_mix : Outport
  wires:
  Tp_phx5/1 -> Mux/1
  Tp_phx6/1 -> Mux/2
  Mux/1 -> Fcn/1
  p_flow_frac/1 -> Mux/3
  Fcn/1 -> Integrator/1
  Integrator/1 -> Tp_phx_mix/1, Mux/4

== system MSDR_v1/HEAT EXCHANGERS/HEAT EXCHANGER LOOP 3/PHX SEC MIXING ==
  Ts_phx5 : Inport
  Ts_phx6 : Inport  Port=2
  s_flow_frac : Inport  Port=3
  Fcn : Fcn  Expr=u[3]*Ws_phx5/ms_phxm*(u[1]-u[4]) + u[3]*Ws_phx6/ms_phxm*(u[2]-u[4])
  Integrator : Integrator  InitialCondition=T0_s_phx1(4)
  Mux : Mux
  Ts_phx_mix : Outport
  wires:
  Ts_phx5/1 -> Mux/1
  Ts_phx6/1 -> Mux/2
  Mux/1 -> Fcn/1
  s_flow_frac/1 -> Mux/3
  Fcn/1 -> Integrator/1
  Integrator/1 -> Ts_phx_mix/1, Mux/4

== system MSDR_v1/HEAT EXCHANGERS/HEAT EXCHANGER LOOP 3/PHX//SHX PUMP ==
  1-D Lookup Table : Lookup_n-D  NumberOfTableDimensions=1  BreakpointsForDimension1=xdat  Table=ydat  InternalRulePriority=Speed  RndMeth=Simplest  InputSameDT=on
  Clock : Clock
  Fcn : Fcn  Expr=exp((1/tau_p)*u)
  Final convection flow rate : Constant  Value=therm_conv
  Scope : Scope
  Subtract : Sum  Inputs=-+
  Switch : Switch  Criteria=u2 > Threshold
  Transport Delay : TransportDelay  DelayTime=10000000  InitialOutput=1
  FLOW FRACTION : Outport
  HEAT TRANSFER FRACTION : Outport  Port=2
  wires:
  Transport Delay/1 -> 1-D Lookup Table/1, Scope/1, FLOW FRACTION/1
  Clock/1 -> Fcn/1
  Switch/1 -> Transport Delay/1
  Fcn/1 -> Subtract/1, Switch/1
  Final convection flow rate/1 -> Subtract/2, Switch/3
  Subtract/1 -> Switch/2
  1-D Lookup Table/1 -> HEAT TRANSFER FRACTION/1

== system MSDR_v1/HEAT EXCHANGERS/HEAT EXCHANGER LOOP 3/PHX5 HEAT TRANSFER ==
  PRIMARY FLUID INLET TEMPERATURE : Inport
  SECONDARY FLUID INLET TEMPERATURE : Inport  Port=2
  PRIMARY FLOW FRACTION : Inport  Port=3
  PRIMARY HEAT TRANSFER FRACTION : Inport  Port=4
  SECONDARY FLOW FRACTION : Inport  Port=5
  SECONDARY HEAT TRANSFER FRACTION : Inport  Port=6
  Mux : Mux  Inputs=16
      settings: DisplayOption=signals
  To Workspace : ToWorkspace  VariableName=phx5_ht  SampleTime=-1
  Tp1_phx5 : Integrator  InitialCondition=T0_p_phx5(1)
  Tp2_phx5 : Integrator  InitialCondition=T0_p_phx5(2)
  "Tp3_phx5 " : Integrator  InitialCondition=T0_p_phx5(3)
  Tp4_phx5 : Integrator  InitialCondition=T0_p_phx5(4)
  Ts1_phx5 : Integrator  InitialCondition=T0_s_phx5(1)
  Ts2_phx5 : Integrator  InitialCondition=T0_s_phx5(2)
  Ts3_phx5 : Integrator  InitialCondition=T0_s_phx5(3)
  Ts4_phx5 : Integrator  InitialCondition=T0_s_phx5(4)
  Tt1_phx5 : Integrator  InitialCondition=T0_t_phx5(1)
  Tt2_phx5 : Integrator  InitialCondition=T0_t_phx5(2)
  d(Tp1_phx5)/dt : Fcn  Expr=(u[13]*Wp_phx5/mp_phx5(1))*(u[1] - u[3]) + (u[14]*hA_p_phx5(1)/mcp_p_phx5(1))*(u[7] - u[3])
  d(Tp2_phx5)/dt : Fcn  Expr=(u[13]*Wp_phx5/mp_phx5(2))*(u[3] - u[4]) + (u[14]*hA_p_phx5(2)/mcp_p_phx5(2))*(u[7] - u[3])
  d(Tp3_phx5)/dt : Fcn  Expr=(u[13]*Wp_phx5/mp_phx5(3))*(u[4] - u[5]) + (u[14]*hA_p_phx5(3)/mcp_p_phx5(3))*(u[8] - u[5])
  d(Tp4_phx5)/dt : Fcn  Expr=(u[13]*Wp_phx5/mp_phx5(4))*(u[5] - u[6]) + (u[14]*hA_p_phx5(4)/mcp_p_phx5(4))*(u[8] - u[5])
  d(Ts1_phx5)/dt : Fcn  Expr=(u[15]*Ws_phx5/ms_phx5(1))*(u[2] - u[9]) + (u[16]*hA_s_phx5(1)/mcp_s_phx5(1))*(u[8] - u[9])
  d(Ts2_phx5)/dt : Fcn  Expr=(u[15]*Ws_phx5/ms_phx5(2))*(u[9] - u[10]) + (u[16]*hA_s_phx5(2)/mcp_s_phx5(2))*(u[8] - u[9])
  d(Ts3_phx5)/dt : Fcn  Expr=(u[15]*Ws_phx5/ms_phx5(3))*(u[10] - u[11]) + (u[16]*hA_s_phx5(3)/mcp_s_phx5(3))*(u[7] - u[11])
  d(Ts4_phx5)/dt : Fcn  Expr=(u[15]*Ws_phx5/ms_phx5(4))*(u[11] - u[12]) + (u[16]*hA_s_phx5(4)/mcp_s_phx5(4))*(u[7] - u[11])
  d(Tt1_phx3)/dt : Fcn  Expr=(u[14]*(hA_p_phx5(1) + hA_p_phx5(2))/mcp_t_phx5(1))*(u[3] - u[7]) + (u[16]*(hA_s_phx5(1) + hA_s_phx5(2))/mcp_t_phx5(1))*(u[11] - u[7])
  d(Tt2_phx5)/dt : Fcn  Expr=(u[14]*(hA_p_phx5(3) + hA_p_phx5(4))/mcp_t_phx5(2))*(u[5] - u[8]) + (u[16]*(hA_s_phx5(3) + hA_s_phx5(4))/mcp_t_phx5(2))*(u[9] - u[8])
  PHX5 TEMPERATURES : Outport
  wires:
  Ts1_phx5/1 -> Mux/9
  Ts2_phx5/1 -> Mux/10
  d(Ts2_phx5)/dt/1 -> Ts2_phx5/1
  d(Tp4_phx5)/dt/1 -> Tp4_phx5/1
  Tt1_phx5/1 -> Mux/7
  d(Tp2_phx5)/dt/1 -> Tp2_phx5/1
  Tp4_phx5/1 -> Mux/6
  d(Tt2_phx5)/dt/1 -> Tt2_phx5/1
  SECONDARY FLUID INLET TEMPERATURE/1 -> Mux/2
  Tt2_phx5/1 -> Mux/8
  Mux/1 -> To Workspace/1, PHX5 TEMPERATURES/1, d(Ts4_phx5)/dt/1, d(Ts3_phx5)/dt/1, d(Ts1_phx5)/dt/1, d(Tt2_phx5)/dt/1, d(Tt1_phx3)/dt/1, d(Tp4_phx5)/dt/1, d(Tp3_phx5)/dt/1, d(Tp2_phx5)/dt/1, d(Tp1_phx5)/dt/1, d(Ts2_phx5)/dt/1
  d(Tp1_phx5)/dt/1 -> Tp1_phx5/1
  d(Ts4_phx5)/dt/1 -> Ts4_phx5/1
  Tp1_phx5/1 -> Mux/3
  d(Ts1_phx5)/dt/1 -> Ts1_phx5/1
  d(Ts3_phx5)/dt/1 -> Ts3_phx5/1
  Ts3_phx5/1 -> Mux/11
  Ts4_phx5/1 -> Mux/12
  "Tp3_phx5 "/1 -> Mux/5
  d(Tp3_phx5)/dt/1 -> "Tp3_phx5 "/1
  Tp2_phx5/1 -> Mux/4
  d(Tt1_phx3)/dt/1 -> Tt1_phx5/1
  PRIMARY FLUID INLET TEMPERATURE/1 -> Mux/1
  PRIMARY FLOW FRACTION/1 -> Mux/13
  PRIMARY HEAT TRANSFER FRACTION/1 -> Mux/14
  SECONDARY FLOW FRACTION/1 -> Mux/15
  SECONDARY HEAT TRANSFER FRACTION/1 -> Mux/16

== system MSDR_v1/HEAT EXCHANGERS/HEAT EXCHANGER LOOP 3/PHX5 MATERIAL TRANSPORT ==
  PHX5 TEMPERATURES : Inport
  wires:
  PHX5 TEMPERATURES/1 -> ?

== system MSDR_v1/HEAT EXCHANGERS/HEAT EXCHANGER LOOP 3/PHX6 HEAT TRANSFER ==
  PRIMARY FLUID INLET TEMPERATURE : Inport
  SECONDARY FLUID INLET TEMPERATURE : Inport  Port=2
  PRIMARY FLOW FRACTION : Inport  Port=3
  PRIMARY HEAT TRANSFER FRACTION : Inport  Port=4
  SECONDARY FLOW FRACTION : Inport  Port=5
  SECONDARY HEAT TRANSFER FRACTION : Inport  Port=6
  Mux : Mux  Inputs=16
      settings: DisplayOption=signals
  To Workspace : ToWorkspace  VariableName=phx6_ht  SampleTime=-1
  Tp1_phx6 : Integrator  InitialCondition=T0_p_phx6(1)
  Tp2_phx6 : Integrator  InitialCondition=T0_p_phx6(2)
  "Tp3_phx6 " : Integrator  InitialCondition=T0_p_phx6(3)
  Tp4_phx6 : Integrator  InitialCondition=T0_p_phx6(4)
  Ts1_phx6 : Integrator  InitialCondition=T0_s_phx6(1)
  Ts2_phx6 : Integrator  InitialCondition=T0_s_phx6(2)
  Ts3_phx6 : Integrator  InitialCondition=T0_s_phx6(3)
  Ts4_phx6 : Integrator  InitialCondition=T0_s_phx6(4)
  Tt1_phx6 : Integrator  InitialCondition=T0_t_phx6(1)
  Tt2_phx6 : Integrator  InitialCondition=T0_t_phx6(2)
  d(Tp1_phx6)/dt : Fcn  Expr=(u[13]*Wp_phx6/mp_phx6(1))*(u[1] - u[3]) + (u[14]*hA_p_phx6(1)/mcp_p_phx6(1))*(u[7] - u[3])
  d(Tp2_phx6)/dt : Fcn  Expr=(u[13]*Wp_phx6/mp_phx6(2))*(u[3] - u[4]) + (u[14]*hA_p_phx6(2)/mcp_p_phx6(2))*(u[7] - u[3])
  d(Tp3_phx6)/dt : Fcn  Expr=(u[13]*Wp_phx6/mp_phx6(3))*(u[4] - u[5]) + (u[14]*hA_p_phx6(3)/mcp_p_phx6(3))*(u[8] - u[5])
  d(Tp4_phx6)/dt : Fcn  Expr=(u[13]*Wp_phx6/mp_phx6(4))*(u[5] - u[6]) + (u[14]*hA_p_phx6(4)/mcp_p_phx6(4))*(u[8] - u[5])
  d(Ts1_phx6)/dt : Fcn  Expr=(u[15]*Ws_phx6/ms_phx6(1))*(u[2] - u[9]) + (u[16]*hA_s_phx6(1)/mcp_s_phx6(1))*(u[8] - u[9])
  d(Ts2_phx6)/dt : Fcn  Expr=(u[15]*Ws_phx6/ms_phx6(2))*(u[9] - u[10]) + (u[16]*hA_s_phx6(2)/mcp_s_phx6(2))*(u[8] - u[9])
  d(Ts3_phx6)/dt : Fcn  Expr=(u[15]*Ws_phx6/ms_phx6(3))*(u[10] - u[11]) + (u[16]*hA_s_phx6(3)/mcp_s_phx6(3))*(u[7] - u[11])
  d(Ts4_phx6)/dt : Fcn  Expr=(u[15]*Ws_phx6/ms_phx6(4))*(u[11] - u[12]) + (u[16]*hA_s_phx6(4)/mcp_s_phx6(4))*(u[7] - u[11])
  d(Tt1_phx6)/dt : Fcn  Expr=(u[14]*(hA_p_phx6(1) + hA_p_phx6(2))/mcp_t_phx6(1))*(u[3] - u[7]) + (u[16]*(hA_s_phx6(1) + hA_s_phx6(2))/mcp_t_phx6(1))*(u[11] - u[7])
  d(Tt2_phx6)/dt : Fcn  Expr=(u[14]*(hA_p_phx6(3) + hA_p_phx6(4))/mcp_t_phx6(2))*(u[5] - u[8]) + (u[16]*(hA_s_phx6(3) + hA_s_phx6(4))/mcp_t_phx6(2))*(u[9] - u[8])
  PHX6 TEMPERATURES : Outport
  wires:
  Ts1_phx6/1 -> Mux/9
  Ts2_phx6/1 -> Mux/10
  d(Ts2_phx6)/dt/1 -> Ts2_phx6/1
  d(Tp4_phx6)/dt/1 -> Tp4_phx6/1
  Tt1_phx6/1 -> Mux/7
  d(Tp2_phx6)/dt/1 -> Tp2_phx6/1
  Tp4_phx6/1 -> Mux/6
  d(Tt2_phx6)/dt/1 -> Tt2_phx6/1
  SECONDARY FLUID INLET TEMPERATURE/1 -> Mux/2
  Tt2_phx6/1 -> Mux/8
  Mux/1 -> To Workspace/1, PHX6 TEMPERATURES/1, d(Ts4_phx6)/dt/1, d(Ts3_phx6)/dt/1, d(Ts1_phx6)/dt/1, d(Tt2_phx6)/dt/1, d(Tt1_phx6)/dt/1, d(Tp4_phx6)/dt/1, d(Tp3_phx6)/dt/1, d(Tp2_phx6)/dt/1, d(Tp1_phx6)/dt/1, d(Ts2_phx6)/dt/1
  d(Tp1_phx6)/dt/1 -> Tp1_phx6/1
  d(Ts4_phx6)/dt/1 -> Ts4_phx6/1
  Tp1_phx6/1 -> Mux/3
  d(Ts1_phx6)/dt/1 -> Ts1_phx6/1
  d(Ts3_phx6)/dt/1 -> Ts3_phx6/1
  Ts3_phx6/1 -> Mux/11
  Ts4_phx6/1 -> Mux/12
  "Tp3_phx6 "/1 -> Mux/5
  d(Tp3_phx6)/dt/1 -> "Tp3_phx6 "/1
  Tp2_phx6/1 -> Mux/4
  d(Tt1_phx6)/dt/1 -> Tt1_phx6/1
  PRIMARY FLUID INLET TEMPERATURE/1 -> Mux/1
  SECONDARY FLOW FRACTION/1 -> Mux/15
  PRIMARY HEAT TRANSFER FRACTION/1 -> Mux/14
  PRIMARY FLOW FRACTION/1 -> Mux/13
  SECONDARY HEAT TRANSFER FRACTION/1 -> Mux/16

== system MSDR_v1/HEAT EXCHANGERS/HEAT EXCHANGER LOOP 3/PHX6 MATERIAL TRANSPORT ==
  PHX6 TEMPERATURES : Inport
  wires:
  PHX6 TEMPERATURES/1 -> ?

== system MSDR_v1/HEAT EXCHANGERS/HEAT EXCHANGER LOOP 3/SHX PRIM MIXING ==
  Tp_shx5 : Inport
  Tp_shx6 : Inport  Port=2
  p_flow_frac : Inport  Port=3
  Fcn : Fcn  Expr=u[3]*Wp_shx5/mp_shxm*(u[1]-u[4]) + u[3]*Wp_shx6/mp_shxm*(u[2]-u[4])
  Integrator : Integrator  InitialCondition=T0_p_shx1(4)
  Mux : Mux
  Tp_shx_mix : Outport
  wires:
  Tp_shx5/1 -> Mux/1
  Tp_shx6/1 -> Mux/2
  Mux/1 -> Fcn/1
  p_flow_frac/1 -> Mux/3
  Fcn/1 -> Integrator/1
  Integrator/1 -> Tp_shx_mix/1, Mux/4

== system MSDR_v1/HEAT EXCHANGERS/HEAT EXCHANGER LOOP 3/SHX SEC MIXING ==
  Ts_shx5 : Inport
  Ts_shx6 : Inport  Port=2
  s_flow_frac : Inport  Port=3
  Fcn : Fcn  Expr=u[3]*Ws_shx5/ms_shxm*(u[1]-u[4]) + u[3]*Ws_shx6/ms_shxm*(u[2]-u[4])
  Integrator : Integrator  InitialCondition=T0_s_shx1(4)
  Mux : Mux
  Ts_shx_mix : Outport
  wires:
  Ts_shx5/1 -> Mux/1
  Ts_shx6/1 -> Mux/2
  Mux/1 -> Fcn/1
  s_flow_frac/1 -> Mux/3
  Fcn/1 -> Integrator/1
  Integrator/1 -> Ts_shx_mix/1, Mux/4

== system MSDR_v1/HEAT EXCHANGERS/HEAT EXCHANGER LOOP 3/SHX//THX PUMP ==
  1-D Lookup Table : Lookup_n-D  NumberOfTableDimensions=1  BreakpointsForDimension1=xdat  Table=ydat  InternalRulePriority=Speed  RndMeth=Simplest  InputSameDT=on
  Clock : Clock
  Fcn : Fcn  Expr=exp((1/tau_p)*u)
  Final convection flow rate : Constant  Value=therm_conv
  Scope : Scope
  Subtract : Sum  Inputs=-+
  Switch : Switch  Criteria=u2 > Threshold
  Transport Delay : TransportDelay  DelayTime=20000000  InitialOutput=1
  FLOW FRACTION : Outport
  HEAT TRANSFER FRACTION : Outport  Port=2
  wires:
  Transport Delay/1 -> 1-D Lookup Table/1, Scope/1, FLOW FRACTION/1
  Clock/1 -> Fcn/1
  Switch/1 -> Transport Delay/1
  Fcn/1 -> Subtract/1, Switch/1
  Final convection flow rate/1 -> Subtract/2, Switch/3
  Subtract/1 -> Switch/2
  1-D Lookup Table/1 -> HEAT TRANSFER FRACTION/1

== system MSDR_v1/HEAT EXCHANGERS/HEAT EXCHANGER LOOP 3/SHX5 HEAT TRANSFER ==
  PRIMARY FLUID INLET TEMPERATURE : Inport
  SECONDARY FLUID INLET TEMPERATURE : Inport  Port=2
  PRIMARY FLOW FRACTION : Inport  Port=3
  PRIMARY HEAT TRANSFER FRACTION : Inport  Port=4
  SECONDARY FLOW FRACTION : Inport  Port=5
  SECONDARY HEAT TRANSFER FRACTION : Inport  Port=6
  Mux : Mux  Inputs=16
      settings: DisplayOption=signals
  To Workspace : ToWorkspace  VariableName=shx5_ht  SampleTime=-1
  Tp1_shx5 : Integrator  InitialCondition=T0_p_shx3(1)
  Tp2_shx5 : Integrator  InitialCondition=T0_p_shx5(2)
  "Tp3_shx5 " : Integrator  InitialCondition=T0_p_shx5(3)
  Tp4_shx5 : Integrator  InitialCondition=T0_p_shx5(4)
  Ts1_shx5 : Integrator  InitialCondition=T0_s_shx5(1)
  Ts2_shx5 : Integrator  InitialCondition=T0_s_shx5(2)
  Ts3_shx5 : Integrator  InitialCondition=T0_s_shx5(3)
  Ts4_shx5 : Integrator  InitialCondition=T0_s_shx5(4)
  Tt1_shx5 : Integrator  InitialCondition=T0_t_shx5(1)
  Tt2_shx5 : Integrator  InitialCondition=T0_t_shx5(2)
  d(Tp1_shx5)/dt : Fcn  Expr=(u[13]*Wp_shx5/mp_shx5(1))*(u[1] - u[3]) + (u[14]*hA_p_shx5(1)/mcp_p_shx5(1))*(u[7] - u[3])
  d(Tp2_shx5)/dt : Fcn  Expr=(u[13]*Wp_shx5/mp_shx5(2))*(u[3] - u[4]) + (u[14]*hA_p_shx5(2)/mcp_p_shx5(2))*(u[7] - u[3])
  d(Tp3_shx5)/dt : Fcn  Expr=(u[13]*Wp_shx5/mp_shx5(3))*(u[4] - u[5]) + (u[14]*hA_p_shx5(3)/mcp_p_shx5(3))*(u[8] - u[5])
  d(Tp4_shx5)/dt : Fcn  Expr=(u[13]*Wp_shx5/mp_shx5(4))*(u[5] - u[6]) + (u[14]*hA_p_shx5(4)/mcp_p_shx5(4))*(u[8] - u[5])
  d(Ts1_shx5)/dt : Fcn  Expr=(u[15]*Ws_shx5/ms_shx5(1))*(u[2] - u[9]) + (u[16]*hA_s_shx5(1)/mcp_s_shx5(1))*(u[8] - u[9])
  d(Ts2_shx5)/dt : Fcn  Expr=(u[15]*Ws_shx5/ms_shx5(2))*(u[9] - u[10]) + (u[16]*hA_s_shx5(2)/mcp_s_shx5(2))*(u[8] - u[9])
  d(Ts3_shx5)/dt : Fcn  Expr=(u[15]*Ws_shx5/ms_shx5(3))*(u[10] - u[11]) + (u[16]*hA_s_shx5(3)/mcp_s_shx5(3))*(u[7] - u[11])
  d(Ts4_shx5)/dt : Fcn  Expr=(u[15]*Ws_shx5/ms_shx5(4))*(u[11] - u[12]) + (u[16]*hA_s_shx5(4)/mcp_s_shx5(4))*(u[7] - u[11])
  d(Tt1_shx5)/dt : Fcn  Expr=(u[14]*(hA_p_shx5(1) + hA_p_shx5(2))/mcp_t_shx5(1))*(u[3] - u[7]) + (u[16]*(hA_s_shx5(1) + hA_s_shx5(2))/mcp_t_shx5(1))*(u[11] - u[7])
  d(Tt2_shx5)/dt : Fcn  Expr=(u[14]*(hA_p_shx5(3) + hA_p_shx5(4))/mcp_t_shx5(2))*(u[5] - u[8]) + (u[16]*(hA_s_shx5(3) + hA_s_shx5(4))/mcp_t_shx5(2))*(u[9] - u[8])
  SHX5 TEMPERATURES : Outport
  wires:
  Ts1_shx5/1 -> Mux/9
  Ts2_shx5/1 -> Mux/10
  d(Ts2_shx5)/dt/1 -> Ts2_shx5/1
  d(Tp4_shx5)/dt/1 -> Tp4_shx5/1
  Tt1_shx5/1 -> Mux/7
  d(Tp2_shx5)/dt/1 -> Tp2_shx5/1
  Tp4_shx5/1 -> Mux/6
  d(Tt2_shx5)/dt/1 -> Tt2_shx5/1
  SECONDARY FLUID INLET TEMPERATURE/1 -> Mux/2
  Tt2_shx5/1 -> Mux/8
  Mux/1 -> To Workspace/1, SHX5 TEMPERATURES/1, d(Ts4_shx5)/dt/1, d(Ts3_shx5)/dt/1, d(Ts2_shx5)/dt/1, d(Ts1_shx5)/dt/1, d(Tt2_shx5)/dt/1, d(Tt1_shx5)/dt/1, d(Tp4_shx5)/dt/1, d(Tp3_shx5)/dt/1, d(Tp2_shx5)/dt/1, d(Tp1_shx5)/dt/1
  d(Tp1_shx5)/dt/1 -> Tp1_shx5/1
  d(Ts4_shx5)/dt/1 -> Ts4_shx5/1
  Tp1_shx5/1 -> Mux/3
  d(Ts1_shx5)/dt/1 -> Ts1_shx5/1
  d(Ts3_shx5)/dt/1 -> Ts3_shx5/1
  Ts3_shx5/1 -> Mux/11
  Ts4_shx5/1 -> Mux/12
  "Tp3_shx5 "/1 -> Mux/5
  d(Tp3_shx5)/dt/1 -> "Tp3_shx5 "/1
  Tp2_shx5/1 -> Mux/4
  d(Tt1_shx5)/dt/1 -> Tt1_shx5/1
  PRIMARY FLUID INLET TEMPERATURE/1 -> Mux/1
  SECONDARY FLOW FRACTION/1 -> Mux/15
  PRIMARY HEAT TRANSFER FRACTION/1 -> Mux/14
  PRIMARY FLOW FRACTION/1 -> Mux/13
  SECONDARY HEAT TRANSFER FRACTION/1 -> Mux/16

== system MSDR_v1/HEAT EXCHANGERS/HEAT EXCHANGER LOOP 3/SHX5 MATERIAL TRANSPORT ==
  SHX5 TEMPERATURES : Inport
  wires:
  SHX5 TEMPERATURES/1 -> ?

== system MSDR_v1/HEAT EXCHANGERS/HEAT EXCHANGER LOOP 3/SHX6 HEAT TRANSFER ==
  PRIMARY FLUID INLET TEMPERATURE : Inport
  SECONDARY FLUID INLET TEMPERATURE : Inport  Port=2
  PRIMARY FLOW FRACTION : Inport  Port=3
  PRIMARY HEAT TRANSFER FRACTION : Inport  Port=4
  SECONDARY FLOW FRACTION : Inport  Port=5
  SECONDARY HEAT TRANSFER FRACTION : Inport  Port=6
  Mux : Mux  Inputs=16
      settings: DisplayOption=signals
  To Workspace : ToWorkspace  VariableName=shx6_ht  SampleTime=-1
  Tp1_shx6 : Integrator  InitialCondition=T0_p_shx6(1)
  Tp2_shx6 : Integrator  InitialCondition=T0_p_shx6(2)
  "Tp3_shx6 " : Integrator  InitialCondition=T0_p_shx6(3)
  Tp4_shx6 : Integrator  InitialCondition=T0_p_shx6(4)
  Ts1_shx6 : Integrator  InitialCondition=T0_s_shx6(1)
  Ts2_shx6 : Integrator  InitialCondition=T0_s_shx6(2)
  Ts3_shx6 : Integrator  InitialCondition=T0_s_shx6(3)
  Ts4_shx6 : Integrator  InitialCondition=T0_s_shx6(4)
  Tt1_shx6 : Integrator  InitialCondition=T0_t_shx6(1)
  Tt2_shx6 : Integrator  InitialCondition=T0_t_shx6(2)
  d(Tp1_shx6)/dt : Fcn  Expr=(u[13]*Wp_shx6/mp_shx6(1))*(u[1] - u[3]) + (u[14]*hA_p_shx6(1)/mcp_p_shx6(1))*(u[7] - u[3])
  d(Tp2_shx6)/dt : Fcn  Expr=(u[13]*Wp_shx6/mp_shx6(2))*(u[3] - u[4]) + (u[14]*hA_p_shx6(2)/mcp_p_shx6(2))*(u[7] - u[3])
  d(Tp3_shx6)/dt : Fcn  Expr=(u[13]*Wp_shx6/mp_shx6(3))*(u[4] - u[5]) + (u[14]*hA_p_shx6(3)/mcp_p_shx6(3))*(u[8] - u[5])
  d(Tp4_shx6)/dt : Fcn  Expr=(u[13]*Wp_shx6/mp_shx6(4))*(u[5] - u[6]) + (u[14]*hA_p_shx6(4)/mcp_p_shx6(4))*(u[8] - u[5])
  d(Ts1_shx6)/dt : Fcn  Expr=(u[15]*Ws_shx6/ms_shx6(1))*(u[2] - u[9]) + (u[16]*hA_s_shx6(1)/mcp_s_shx6(1))*(u[8] - u[9])
  d(Ts2_shx6)/dt : Fcn  Expr=(u[15]*Ws_shx6/ms_shx6(2))*(u[9] - u[10]) + (u[16]*hA_s_shx6(2)/mcp_s_shx6(2))*(u[8] - u[9])
  d(Ts3_shx6)/dt : Fcn  Expr=(u[15]*Ws_shx6/ms_shx6(3))*(u[10] - u[11]) + (u[16]*hA_s_shx6(3)/mcp_s_shx6(3))*(u[7] - u[11])
  d(Ts4_shx4)/dt : Fcn  Expr=(u[15]*Ws_shx6/ms_shx6(4))*(u[11] - u[12]) + (u[16]*hA_s_shx6(4)/mcp_s_shx6(4))*(u[7] - u[11])
  d(Tt1_shx6)/dt : Fcn  Expr=(u[14]*(hA_p_shx6(1) + hA_p_shx6(2))/mcp_t_shx6(1))*(u[3] - u[7]) + (u[16]*(hA_s_shx6(1) + hA_s_shx6(2))/mcp_t_shx6(1))*(u[11] - u[7])
  d(Tt2_shx6)/dt : Fcn  Expr=(u[14]*(hA_p_shx6(3) + hA_p_shx6(4))/mcp_t_shx6(2))*(u[5] - u[8]) + (u[16]*(hA_s_shx6(3) + hA_s_shx6(4))/mcp_t_shx6(2))*(u[9] - u[8])
  SHX6 TEMPERATURES : Outport
  wires:
  Ts1_shx6/1 -> Mux/9
  Ts2_shx6/1 -> Mux/10
  d(Ts2_shx6)/dt/1 -> Ts2_shx6/1
  d(Tp4_shx6)/dt/1 -> Tp4_shx6/1
  Tt1_shx6/1 -> Mux/7
  d(Tp2_shx6)/dt/1 -> Tp2_shx6/1
  Tp4_shx6/1 -> Mux/6
  d(Tt2_shx6)/dt/1 -> Tt2_shx6/1
  SECONDARY FLUID INLET TEMPERATURE/1 -> Mux/2
  Tt2_shx6/1 -> Mux/8
  Mux/1 -> To Workspace/1, SHX6 TEMPERATURES/1, d(Ts4_shx4)/dt/1, d(Ts3_shx6)/dt/1, d(Ts2_shx6)/dt/1, d(Ts1_shx6)/dt/1, d(Tt2_shx6)/dt/1, d(Tt1_shx6)/dt/1, d(Tp4_shx6)/dt/1, d(Tp3_shx6)/dt/1, d(Tp2_shx6)/dt/1, d(Tp1_shx6)/dt/1
  d(Tp1_shx6)/dt/1 -> Tp1_shx6/1
  d(Ts4_shx4)/dt/1 -> Ts4_shx6/1
  Tp1_shx6/1 -> Mux/3
  d(Ts1_shx6)/dt/1 -> Ts1_shx6/1
  d(Ts3_shx6)/dt/1 -> Ts3_shx6/1
  Ts3_shx6/1 -> Mux/11
  Ts4_shx6/1 -> Mux/12
  "Tp3_shx6 "/1 -> Mux/5
  d(Tp3_shx6)/dt/1 -> "Tp3_shx6 "/1
  Tp2_shx6/1 -> Mux/4
  d(Tt1_shx6)/dt/1 -> Tt1_shx6/1
  PRIMARY FLUID INLET TEMPERATURE/1 -> Mux/1
  SECONDARY FLOW FRACTION/1 -> Mux/15
  PRIMARY HEAT TRANSFER FRACTION/1 -> Mux/14
  PRIMARY FLOW FRACTION/1 -> Mux/13
  SECONDARY HEAT TRANSFER FRACTION/1 -> Mux/16

== system MSDR_v1/HEAT EXCHANGERS/HEAT EXCHANGER LOOP 3/SHX6 MATERIAL TRANSPORT ==
  SHX6 TEMPERATURES : Inport
  wires:
  SHX6 TEMPERATURES/1 -> ?
